simulink model "control"  (R2018b)
settings: Solver=FixedStepDiscrete  StartTime=0.0  StopTime=inf  FixedStep=1/400  RelTol=1e-3
undefined symbols (not defined in the file): conf
libraries: libnng x1, sldrtlib x1
settings Model: Creator=petrb  LastModifiedBy=Lenovo
settings SolverCC: PositivePriorityOrder=on
settings OptimizationCC: PassReuseOutputArgsAs=Individual arguments  MaxStackSize=64
settings DebuggingCC: ParameterTunabilityLossMsg=error  LibraryContextMissingDiagnostic=none
settings HardwareCC: ProdBitPerPointer=32  ProdBitPerSizeT=32  ProdBitPerPtrDiffT=32  ProdLargestAtomicInteger=Long  ProdLargestAtomicFloat=Double  ProdWordSize=32  ProdHWDeviceType=ARM Compatible->ARM Cortex
settings SFSimCC: SimUseLocalCustomCode=off  MATLABDynamicMemAlloc=off
settings RTWCC: SystemTargetFile=ert.tlc  HardwareBoard=BeagleBone Blue  TLCOptions="-aInlineSetEventsForThisBaseRateFcn=TLC_FALSE -aSuppressMultiTaskScheduler=TLC_FALSE  -aRateBasedStepFcn=0"  TemplateMakefile=ert_default_tmf  RTWUseLocalCustomCode=off  RTWUseSimCustomCode=on  Toolchain=GNU GCC BeagleBone Blue  IncludeHyperlinkInReport=on
settings CodeAppCC: ForceParamTrailComments=on  IgnoreCustomStorageClasses=off  OperatorAnnotations=on  SimulinkDataObjDesc=on  SFDataObjDesc=on  InsertBlockDesc=on
settings ERTTargetCC: SupportNonInlinedSFcns=on  SupportVariableSizeSignals=on

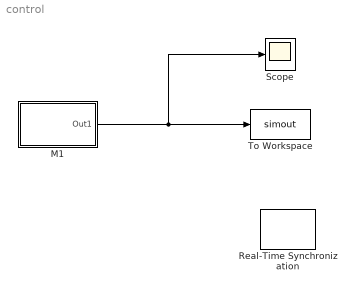
== system control ==
  M1 : Subsystem
  Real-Time Synchronization : sldrtlib/Real-Time Synchronization  SampleTime=conf.CommsBackend.SampleTime  MaxMissedTicks=40402  ShowMissedTicks=off  YieldWhenWaiting=on
  Scope : Scope
  To Workspace : ToWorkspace  VariableName=simout  SaveFormat=Timeseries  SampleTime=-1
  wires:
  M1/1(Out1) -> Scope/1, To Workspace/1

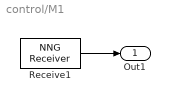
== system control/M1 ==
  Receive1 : libnng/NNG Receiver  hosturl='tcp://192.168.88.18:25500'  sampletime=0.005  datawidth=3
  Out1 : Outport
  wires:
  Receive1/1 -> Out1/1
